simulink model "qdqd_robot"  (R2022b)
settings: Solver=FixedStepAuto  StartTime=0.0  StopTime=10  FixedStep=0.01  RelTol=1e-3
model workspace: external: MATLAB File C:\Users\Tin\Desktop\tailieuhoc\TT Robotics\task2\robot_DataFile2.m (data not in the file)
undefined symbols (not defined in the file or in its folder): smiData, X, Y, Z
libraries: sm_lib x21, nesl_utility x4
settings Model: Creator=Tin  LastModifiedBy=Tin

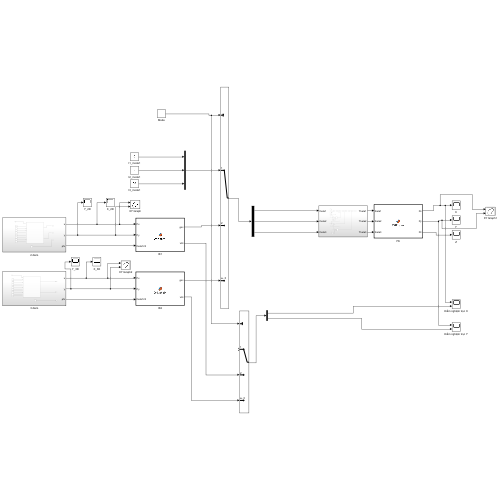
[thumbnail: Simulink's stored preview of the top-level diagram]
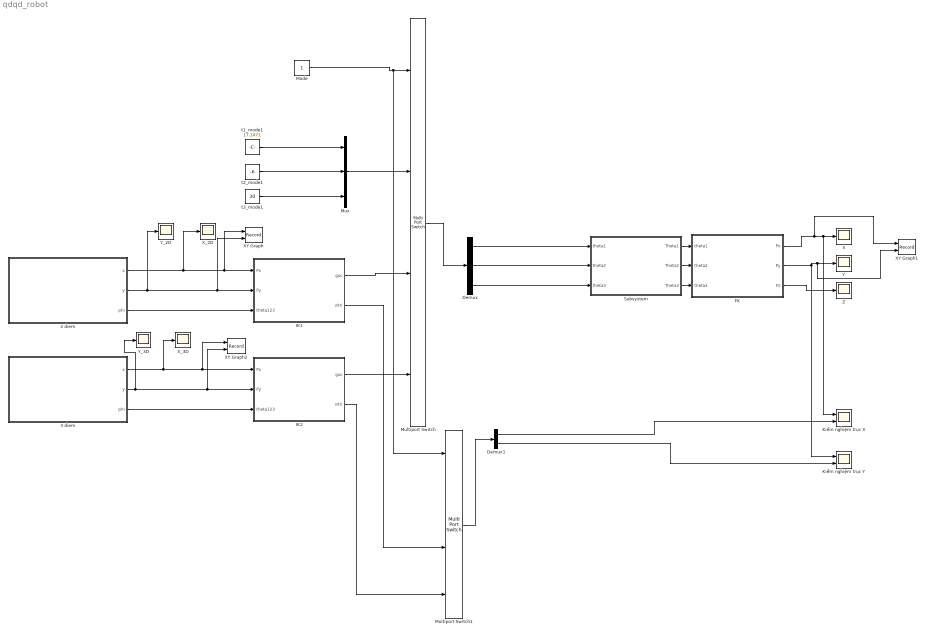
== system qdqd_robot ==
  2 diem : Subsystem
  3 diem : Subsystem
  Demux : Demux  Outputs=3
  Demux1 : Demux  Outputs=2
  FK : MATLAB Function  TreatAsAtomicUnit=on
  IK1 : MATLAB Function  TreatAsAtomicUnit=on
  IK2 : MATLAB Function  TreatAsAtomicUnit=on
  Kiểm nghiệm trục X : Scope  NumInputPorts=2
  Kiểm nghiệm trục Y : Scope  NumInputPorts=2
  Mode : Constant
  Multiport Switch : MultiPortSwitch  SaturateOnIntegerOverflow=off  InputSameDT=off
  Multiport Switch1 : MultiPortSwitch  SaturateOnIntegerOverflow=off  InputSameDT=off
  Mux : Mux  Inputs=3
  Subsystem : Subsystem
  X : Scope
  XY Graph : Record  FileSettingsInternal="{\"entries\":[{\"content\":{\"excelSettings\":{\"content\":{},\"type\":\"Streamout.ExcelSettings\"}},\"type\":\"Streamout.FileSettingStorage\",\"uuid\":\"97201033-76aa-4202-b919-b78145d5e60c\"}],\"packageUris\":[\"http://schema.mathworks.com/mf0/streamout_blocks/R2020a\"],\"version\":\"1.0\"}"  Layout=[1 1]  SignalsInternal="{\"entries\":[{\"content\":{\"signals\":[{\"content\":{\"blockPath\":[\"qdqd_robot/XY Graph\"],\"channel\":[],\"dimensions\":[1],\"domain\":\"qdqd_robot/XY Graph\",\"lineColor\":\"#a2142f\",\"plots\":[1],\"port\":1,\"sid\":[\"\"],\"signalID\":186,\"signalName\":\"2 diem:1\"},\"type\":\"RecordBlkView.Signal\",\"uuid\":\"08513785-76e9-4c55-b008-f54bb21082a6\"},{\"content\":{\"blockPath\":[\"qdqd_robot/XY Graph\"],\"channel\":[],\"dimensions\":[1],\"domain\":\"qdqd_robot/XY Graph\",\"lineColor\":\"#139fff\",\"plots\":[1],\"port\":2,\"sid\":[\"\"],\"signalID\":190,\"signalName\":\"2 diem:2\"},\"type\":\"RecordBlkView.Signal\",\"uuid\":\"6af3ea91-2b2f-4a9b-90b3-e45fbf568ca8\"}]},\"type\":\"RecordBlkView.InputSignals\",\"uuid\":\"c4f7b2ae-604a-40bb-aba8-63fb868da412\"}],\"packageUris\":[\"http://schema.mathworks.com/mf0/streamout_blocks/R2020a\"],\"version\":\"1.0\"}"  VisualizationBindings="{\"xyplotplugin\":{\"info\":[{\"series\":[{\"bindingParametersList\":[{\"parameter\":\"X-Axis\",\"signalID\":186,\"signalName\":\"2 diem:1\"},{\"parameter\":\"Y-Axis\",\"signalID\":190,\"signalName\":\"2 diem:2\"}],\"seriesID\":19907}],\"subplotID\":1}]}}"  CompatibilityTag=XY
  XY Graph1 : Record  FileSettingsInternal="{\"entries\":[{\"content\":{\"excelSettings\":{\"content\":{},\"type\":\"Streamout.ExcelSettings\"}},\"type\":\"Streamout.FileSettingStorage\",\"uuid\":\"ef5a2e5f-ada7-4355-a35d-416917ef2084\"}],\"packageUris\":[\"http://schema.mathworks.com/mf0/streamout_blocks/R2020a\"],\"version\":\"1.0\"}"  Layout=[1 1]  SignalsInternal="{\"entries\":[{\"content\":{\"signals\":[{\"content\":{\"blockPath\":[\"qdqd_robot/XY Graph1\"],\"channel\":[],\"dimensions\":[1],\"domain\":\"qdqd_robot/XY Graph1\",\"lineColor\":\"#a2142f\",\"plots\":[1],\"port\":1,\"sid\":[\"\"],\"signalID\":194,\"signalName\":\"FK:1\"},\"type\":\"RecordBlkView.Signal\",\"uuid\":\"117ca86f-aa11-44ab-9443-b09f4f7bf889\"},{\"content\":{\"blockPath\":[\"qdqd_robot/XY Graph1\"],\"channel\":[],\"dimensions\":[1],\"domain\":\"qdqd_robot/XY Graph1\",\"lineColor\":\"#139fff\",\"plots\":[1],\"port\":2,\"sid\":[\"\"],\"signalID\":198,\"signalName\":\"FK:2\"},\"type\":\"RecordBlkView.Signal\",\"uuid\":\"99251a9f-89e7-4e57-8cb5-748fe57cbdd2\"}]},\"type\":\"RecordBlkView.InputSignals\",\"uuid\":\"e90fa3b0-753d-4f20-842e-d0b0260bec66\"}],\"packageUris\":[\"http://schema.mathworks.com/mf0/streamout_blocks/R2020a\"],\"version\":\"1.0\"}"  VisualizationBindings="{\"xyplotplugin\":{\"info\":[{\"series\":[{\"bindingParametersList\":[{\"parameter\":\"X-Axis\",\"signalID\":194,\"signalName\":\"FK:1\"},{\"parameter\":\"Y-Axis\",\"signalID\":198,\"signalName\":\"FK:2\"}],\"seriesID\":49500}],\"subplotID\":1}]}}"  CompatibilityTag=XY
  XY Graph2 : Record  FileSettingsInternal="{\"entries\":[{\"content\":{\"excelSettings\":{\"content\":{},\"type\":\"Streamout.ExcelSettings\"}},\"type\":\"Streamout.FileSettingStorage\",\"uuid\":\"42d82971-a484-44fd-ac3b-312511253240\"}],\"packageUris\":[\"http://schema.mathworks.com/mf0/streamout_blocks/R2020a\"],\"version\":\"1.0\"}"  Layout=[1 1]  SignalsInternal="{\"entries\":[{\"content\":{\"signals\":[{\"content\":{\"blockPath\":[\"qdqd_robot/XY Graph2\"],\"channel\":[],\"dimensions\":[1],\"domain\":\"qdqd_robot/XY Graph2\",\"lineColor\":\"#a2142f\",\"plots\":[1],\"port\":1,\"sid\":[\"\"],\"signalID\":202,\"signalName\":\"3 diem:1\"},\"type\":\"RecordBlkView.Signal\",\"uuid\":\"d0b55c77-b964-4692-b3b0-299111d60012\"},{\"content\":{\"blockPath\":[\"qdqd_robot/XY Graph2\"],\"channel\":[],\"dimensions\":[1],\"domain\":\"qdqd_robot/XY Graph2\",\"lineColor\":\"#139fff\",\"plots\":[1],\"port\":2,\"sid\":[\"\"],\"signalID\":206,\"signalName\":\"3 diem:2\"},\"type\":\"RecordBlkView.Signal\",\"uuid\":\"4c5f2143-5546-468c-9f3f-87db4ee2b5a3\"}]},\"type\":\"RecordBlkView.InputSignals\",\"uuid\":\"6f2205dc-2759-4ab6-9096-b1192ef20588\"}],\"packageUris\":[\"http://schema.mathworks.com/mf0/streamout_blocks/R2020a\"],\"version\":\"1.0\"}"  VisualizationBindings="{\"xyplotplugin\":{\"info\":[{\"series\":[{\"bindingParametersList\":[{\"parameter\":\"X-Axis\",\"signalID\":202,\"signalName\":\"3 diem:1\"},{\"parameter\":\"Y-Axis\",\"signalID\":206,\"signalName\":\"3 diem:2\"}],\"seriesID\":60577}],\"subplotID\":1}]}}"  CompatibilityTag=XY
  X_2D : Scope
  X_3D : Scope
  Y : Scope
  Y_2D : Scope
  Y_3D : Scope
  Z : Scope
  t1_mode1 : Constant  Value=17.1471
  t2_mode1 : Constant  Value=-6
  t3_mode1 : Constant  Value=30
  wires:
  2 diem/3(phi) -> IK1/3(theta123)
  2 diem/2(y) -> Y_2D/1, IK1/2(Py), XY Graph/2
  3 diem/3(phi) -> IK2/3(theta123)
  IK2/1(goc) -> Multiport Switch/4
  t2_mode1/1 -> Mux/2
  t3_mode1/1 -> Mux/3
  Mux/1 -> Multiport Switch/2
  Demux/2 -> Subsystem/2(theta2)
  Demux/3 -> Subsystem/3(theta3)
  Multiport Switch/1 -> Demux/1
  t1_mode1/1 -> Mux/1
  3 diem/2(y) -> Y_3D/1, IK2/2(Py), XY Graph2/2
  3 diem/1(x) -> IK2/1(Px), XY Graph2/1, X_3D/1
  IK1/1(goc) -> Multiport Switch/3
  Subsystem/1(Theta1) -> FK/1(theta1)
  Subsystem/2(Theta2) -> FK/2(theta2)
  Subsystem/3(Theta3) -> FK/3(theta3)
  FK/1(Px) -> XY Graph1/1, Kiểm nghiệm trục X/1, X/1
  FK/2(Py) -> XY Graph1/2, Y/1, Kiểm nghiệm trục Y/1
  FK/3(Pz) -> Z/1
  Demux/1 -> Subsystem/1(theta1)
  2 diem/1(x) -> IK1/1(Px), XY Graph/1, X_2D/1
  Mode/1 -> Multiport Switch1/1, Multiport Switch/1
  IK1/2(vitri) -> Multiport Switch1/3
  IK2/2(vitri) -> Multiport Switch1/4
  Multiport Switch1/1 -> Demux1/1
  Demux1/1 -> Kiểm nghiệm trục X/2
  Demux1/2 -> Kiểm nghiệm trục Y/2

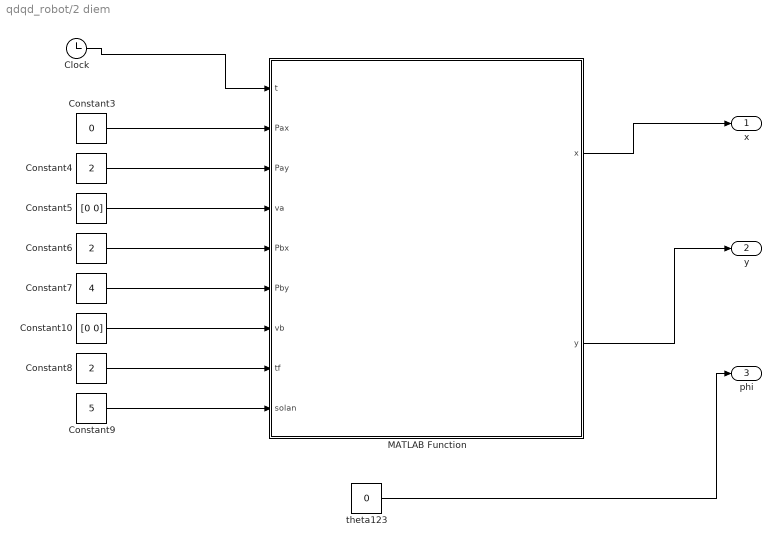
== system qdqd_robot/2 diem ==
  Clock : Clock
  Constant10 : Constant  Value=[0 0]
  Constant3 : Constant  Value=0
  Constant4 : Constant  Value=2
  Constant5 : Constant  Value=[0 0]
  Constant6 : Constant  Value=2
  Constant7 : Constant  Value=4
  Constant8 : Constant  Value=2
  Constant9 : Constant  Value=5
  MATLAB Function : MATLAB Function  TreatAsAtomicUnit=on
  theta123 : Constant  Value=0
  x : Outport
  y : Outport  Port=2
  phi : Outport  Port=3
  wires:
  Constant6/1 -> MATLAB Function/5(Pbx)
  Constant3/1 -> MATLAB Function/2(Pax)
  Constant7/1 -> MATLAB Function/6(Pby)
  Clock/1 -> MATLAB Function/1(t)
  Constant8/1 -> MATLAB Function/8(tf)
  Constant9/1 -> MATLAB Function/9(solan)
  Constant10/1 -> MATLAB Function/7(vb)
  Constant5/1 -> MATLAB Function/4(va)
  Constant4/1 -> MATLAB Function/3(Pay)
  MATLAB Function/1(x) -> x/1
  theta123/1 -> phi/1
  MATLAB Function/2(y) -> y/1

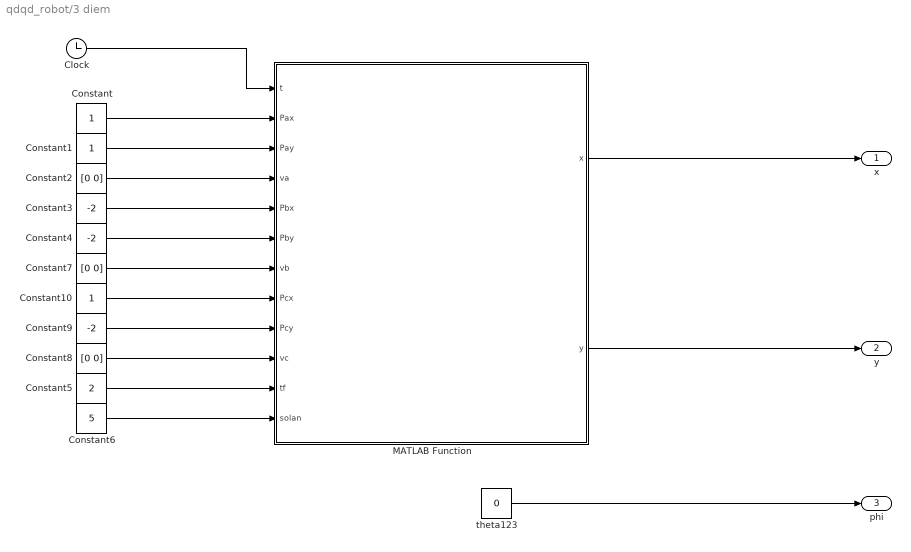
== system qdqd_robot/3 diem ==
  Clock : Clock
      settings: Decimation=30
  Constant : Constant
  Constant1 : Constant
  Constant10 : Constant
  Constant2 : Constant  Value=[0 0]
  Constant3 : Constant  Value=-2
  Constant4 : Constant  Value=-2
  Constant5 : Constant  Value=2
  Constant6 : Constant  Value=5
  Constant7 : Constant  Value=[0 0]
  Constant8 : Constant  Value=[0 0]
  Constant9 : Constant  Value=-2
  MATLAB Function : MATLAB Function  TreatAsAtomicUnit=on
  theta123 : Constant  Value=0
  x : Outport
  y : Outport  Port=2
  phi : Outport  Port=3
  wires:
  theta123/1 -> phi/1
  Constant10/1 -> MATLAB Function/8(Pcx)
  Constant9/1 -> MATLAB Function/9(Pcy)
  Constant3/1 -> MATLAB Function/5(Pbx)
  Constant8/1 -> MATLAB Function/10(vc)
  Constant5/1 -> MATLAB Function/11(tf)
  Constant/1 -> MATLAB Function/2(Pax)
  Constant2/1 -> MATLAB Function/4(va)
  Clock/1 -> MATLAB Function/1(t)
  Constant4/1 -> MATLAB Function/6(Pby)
  Constant1/1 -> MATLAB Function/3(Pay)
  Constant7/1 -> MATLAB Function/7(vb)
  Constant6/1 -> MATLAB Function/12(solan)
  MATLAB Function/1(x) -> x/1
  MATLAB Function/2(y) -> y/1

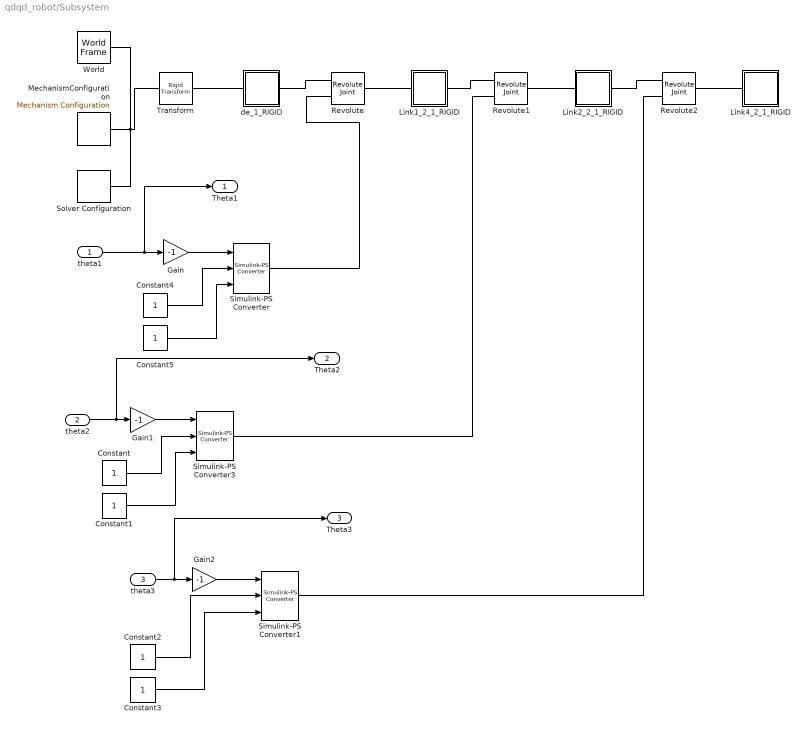
== system qdqd_robot/Subsystem ==
  theta1 : Inport
  theta2 : Inport  Port=2
  theta3 : Inport  Port=3
  Constant{,1..5} (6 alike) : Constant
  Gain : Gain  Gain=-1
  Gain1 : Gain  Gain=-1
  Gain2 : Gain  Gain=-1
  Link1_2_1_RIGID : Subsystem
  Link2_2_1_RIGID : Subsystem
  Link4_2_1_RIGID : Subsystem
  MechanismConfiguration : sm_lib/Utilities/Mechanism Configuration  UniformGravity=Constant  GravityVector=[0 -9.80665 0]  GravityUnits=m/s^2  LinearizationDelta=0.001  JointModeTransitionNonlinearIterations=2
  Revolute : sm_lib/Joints/Revolute Joint  JointMode=Normal  SenseConstraintForce=off  SenseConstraintForceX=off  SenseConstraintForceY=off  SenseConstraintForceZ=off  SenseConstraintTorque=off  SenseConstraintTorqueX=off  SenseConstraintTorqueY=off  SenseConstraintTorqueZ=off  SenseTotalForce=off  SenseTotalForceX=off  SenseTotalForceY=off  SenseTotalForceZ=off  SenseTotalTorque=off  SenseTotalTorqueX=off  SenseTotalTorqueY=off  SenseTotalTorqueZ=off  CompositeWrenchDir=FollowerOnBase  CompositeWrenchFrame=BaseFrame  EquilibriumPosition=0  EquilibriumPositionUnits=deg  SpringStiffness=0  SpringStiffnessUnits=N*m/deg  DampingCoefficient=0  DampingCoefficientUnits=N*m/(deg/s)  TorqueActuationMode=ComputedTorque  MotionActuationMode=InputMotion  SensePosition=off  SenseVelocity=off  SenseAcceleration=off  SenseTorqueForce=off  SenseLowerLimitTorqueForce=off  SenseUpperLimitTorqueForce=off  LowerLimitSpecify=off  LowerLimitBound=-90  LowerLimitBoundUnits=deg  LowerLimitStiffness=1e4  LowerLimitStiffnessUnits=N*m/deg  LowerLimitDamping=10  LowerLimitDampingUnits=N*m/(deg/s)  LowerLimitTransitionRegionWidth=0.1  LowerLimitTransitionRegionWidthUnits=deg  UpperLimitSpecify=off  UpperLimitBound=90  UpperLimitBoundUnits=deg  UpperLimitStiffness=1e4  UpperLimitStiffnessUnits=N*m/deg  UpperLimitDamping=10  UpperLimitDampingUnits=N*m/(deg/s)  UpperLimitTransitionRegionWidth=0.1  UpperLimitTransitionRegionWidthUnits=deg  PositionTargetSpecify=on  PositionTargetPriority=Low  PositionTargetValue=smiData.RevoluteJoint(1).Rz.Pos  PositionTargetValueUnits=deg  VelocityTargetSpecify=off  VelocityTargetPriority=High  VelocityTargetValue=0  VelocityTargetValueUnits=deg/s
  Revolute1 : sm_lib/Joints/Revolute Joint  JointMode=Normal  SenseConstraintForce=off  SenseConstraintForceX=off  SenseConstraintForceY=off  SenseConstraintForceZ=off  SenseConstraintTorque=off  SenseConstraintTorqueX=off  SenseConstraintTorqueY=off  SenseConstraintTorqueZ=off  SenseTotalForce=off  SenseTotalForceX=off  SenseTotalForceY=off  SenseTotalForceZ=off  SenseTotalTorque=off  SenseTotalTorqueX=off  SenseTotalTorqueY=off  SenseTotalTorqueZ=off  CompositeWrenchDir=FollowerOnBase  CompositeWrenchFrame=BaseFrame  EquilibriumPosition=0  EquilibriumPositionUnits=deg  SpringStiffness=0  SpringStiffnessUnits=N*m/deg  DampingCoefficient=0  DampingCoefficientUnits=N*m/(deg/s)  TorqueActuationMode=ComputedTorque  MotionActuationMode=InputMotion  SensePosition=off  SenseVelocity=off  SenseAcceleration=off  SenseTorqueForce=off  SenseLowerLimitTorqueForce=off  SenseUpperLimitTorqueForce=off  LowerLimitSpecify=off  LowerLimitBound=-90  LowerLimitBoundUnits=deg  LowerLimitStiffness=1e4  LowerLimitStiffnessUnits=N*m/deg  LowerLimitDamping=10  LowerLimitDampingUnits=N*m/(deg/s)  LowerLimitTransitionRegionWidth=0.1  LowerLimitTransitionRegionWidthUnits=deg  UpperLimitSpecify=off  UpperLimitBound=90  UpperLimitBoundUnits=deg  UpperLimitStiffness=1e4  UpperLimitStiffnessUnits=N*m/deg  UpperLimitDamping=10  UpperLimitDampingUnits=N*m/(deg/s)  UpperLimitTransitionRegionWidth=0.1  UpperLimitTransitionRegionWidthUnits=deg  PositionTargetSpecify=on  PositionTargetPriority=Low  PositionTargetValue=smiData.RevoluteJoint(2).Rz.Pos  PositionTargetValueUnits=deg  VelocityTargetSpecify=off  VelocityTargetPriority=High  VelocityTargetValue=0  VelocityTargetValueUnits=deg/s
  Revolute2 : sm_lib/Joints/Revolute Joint  JointMode=Normal  SenseConstraintForce=off  SenseConstraintForceX=off  SenseConstraintForceY=off  SenseConstraintForceZ=off  SenseConstraintTorque=off  SenseConstraintTorqueX=off  SenseConstraintTorqueY=off  SenseConstraintTorqueZ=off  SenseTotalForce=off  SenseTotalForceX=off  SenseTotalForceY=off  SenseTotalForceZ=off  SenseTotalTorque=off  SenseTotalTorqueX=off  SenseTotalTorqueY=off  SenseTotalTorqueZ=off  CompositeWrenchDir=FollowerOnBase  CompositeWrenchFrame=BaseFrame  EquilibriumPosition=0  EquilibriumPositionUnits=deg  SpringStiffness=0  SpringStiffnessUnits=N*m/deg  DampingCoefficient=0  DampingCoefficientUnits=N*m/(deg/s)  TorqueActuationMode=ComputedTorque  MotionActuationMode=InputMotion  SensePosition=off  SenseVelocity=off  SenseAcceleration=off  SenseTorqueForce=off  SenseLowerLimitTorqueForce=off  SenseUpperLimitTorqueForce=off  LowerLimitSpecify=off  LowerLimitBound=-90  LowerLimitBoundUnits=deg  LowerLimitStiffness=1e4  LowerLimitStiffnessUnits=N*m/deg  LowerLimitDamping=10  LowerLimitDampingUnits=N*m/(deg/s)  LowerLimitTransitionRegionWidth=0.1  LowerLimitTransitionRegionWidthUnits=deg  UpperLimitSpecify=off  UpperLimitBound=90  UpperLimitBoundUnits=deg  UpperLimitStiffness=1e4  UpperLimitStiffnessUnits=N*m/deg  UpperLimitDamping=10  UpperLimitDampingUnits=N*m/(deg/s)  UpperLimitTransitionRegionWidth=0.1  UpperLimitTransitionRegionWidthUnits=deg  PositionTargetSpecify=on  PositionTargetPriority=Low  PositionTargetValue=smiData.RevoluteJoint(3).Rz.Pos  PositionTargetValueUnits=deg  VelocityTargetSpecify=off  VelocityTargetPriority=High  VelocityTargetValue=0  VelocityTargetValueUnits=deg/s
  Simulink-PS Converter : nesl_utility/Simulink-PS Converter  PhysicalDomain=network_engine_domain  SubClassName=ps_input  LeftPortType=input  RightPortType=output  PseudoPeriodic=off  Frequencies=[]  NoiseDistribution=none  NoiseParameters=[]  Unit=1  AffineConversion=on  FilteringAndDerivatives=provide  SimscapeFilterOrder=2  InputFilterTimeConstant=0.001  UdotUserProvided=2
  Simulink-PS Converter1 : nesl_utility/Simulink-PS Converter  PhysicalDomain=network_engine_domain  SubClassName=ps_input  LeftPortType=input  RightPortType=output  PseudoPeriodic=off  Frequencies=[]  NoiseDistribution=none  NoiseParameters=[]  Unit=1  AffineConversion=on  FilteringAndDerivatives=provide  SimscapeFilterOrder=2  InputFilterTimeConstant=0.001  UdotUserProvided=2
  Simulink-PS Converter3 : nesl_utility/Simulink-PS Converter  PhysicalDomain=network_engine_domain  SubClassName=ps_input  LeftPortType=input  RightPortType=output  PseudoPeriodic=off  Frequencies=[]  NoiseDistribution=none  NoiseParameters=[]  Unit=1  AffineConversion=on  FilteringAndDerivatives=provide  SimscapeFilterOrder=2  InputFilterTimeConstant=0.001  UdotUserProvided=2
  Solver Configuration : nesl_utility/Solver Configuration  PhysicalDomain=network_engine_domain  SubClassName=solver  LeftPortType=input  RightPortType=generic  Tones=[]  Harmonics=[]  SimulateNoise=off  Profile=off  UseLocalSampling=off  EnableSwitchedLinearOptims=on  FrequencyDomain=off  UseCCode=off  RelTol=0.001  AbsTol=0.001  MinStep=1e-09  ToWorkspace=off  RevertToSquareIcSolve=off  NumHomotopyIterations=100  PhasorMode=off  PhasorModeNumHarmonics=1  ConsistencySolver=NEWTON_XTOL_AFTER_FTOL  IndexReductionMethod=DerivativeReplacement  DoDC=off  ResidualTolerance=1e-09  ConsistencyTolSource=GLOBAL  ConsistencyAbsTol=0.001  ConsistencyRelTol=0.001  ConsistencyTolFactor=0.001  UseLocalSolver=off  LocalSolverChoice=NE_BACKWARD_EULER_ADVANCER  ResolveIndetEquations=on  FunctionEvalNumThread=1  LocalSolverSampleTime=0.001  DoFixedCost=off  MaxNonlinIter=3  MaxModeIter=2  ComputeImpulses=off  ImpulseIterations=2  LinearAlgebra=auto  LinearAlgebraNumThread=0  EquationFormulation=NE_TIME_EF  DelaysMemoryBudget=1024  AutomaticFiltering=on  FilteringTimeConstant=0.001  PartitionStorageMethod=AS_NEEDED  PartitionMemoryBudget=1024  PartitionMethod=ROBUST
  Transform : sm_lib/Frames and Transforms/Rigid Transform  TranslationMethod=Cartesian  TranslationStandardOffset=0  TranslationLengthUnit=mm  TranslationStandardAxis=+Z  TranslationCartesianOffset=smiData.RigidTransform(2).translation  TranslationROffset=0  TranslationROffsetUnits=m  TranslationZOffset=0  TranslationZOffsetUnits=m  TranslationThetaOffset=0  TranslationThetaOffsetUnits=deg  RotationMethod=ArbitraryAxis  RotationAngleUnits=rad  RotationStandardAxis=+Z  RotationAngle=smiData.RigidTransform(2).angle  RotationArbitraryAxis=smiData.RigidTransform(2).axis  FollAlignAxisA=+X  BaseAlignAxisA=+Y  FollAlignAxisB=+Y  BaseAlignAxisB=+Z  RotationSequenceAxes=FollowerAxes  RotationSequence=XYX  RotationSequenceAngles=[0 0 0]  RotationSequenceAnglesUnits=deg  RotationMatrix=[1 0 0; 0 1 0; 0 0 1]  Quaternion=[1 0 0 0]
  World : sm_lib/Frames and Transforms/World Frame
  de_1_RIGID : Subsystem
  Theta1 : Outport
  Theta2 : Outport  Port=2
  Theta3 : Outport  Port=3
  wires:
  theta2/1 -> Theta2/1, Gain1/1
  Gain1/1 -> Simulink-PS Converter3/1
  Gain2/1 -> Simulink-PS Converter1/1
  theta3/1 -> Theta3/1, Gain2/1
  Constant/1 -> Simulink-PS Converter3/2
  Constant1/1 -> Simulink-PS Converter3/3
  Constant2/1 -> Simulink-PS Converter1/2
  Constant3/1 -> Simulink-PS Converter1/3
  Constant4/1 -> Simulink-PS Converter/2
  Constant5/1 -> Simulink-PS Converter/3
  Gain/1 -> Simulink-PS Converter/1
  theta1/1 -> Theta1/1, Gain/1
  connections:
  World/RConn1 -- MechanismConfiguration/RConn1 -- Solver Configuration/RConn1 -- Transform/LConn1
  Simulink-PS Converter/RConn1 -- Revolute/LConn2
  Link1_2_1_RIGID/LConn1 -- Revolute/RConn1
  Link2_2_1_RIGID/RConn1 -- Revolute2/LConn1
  Transform/RConn1 -- de_1_RIGID/LConn1
  Link2_2_1_RIGID/LConn1 -- Revolute1/RConn1
  Link4_2_1_RIGID/LConn1 -- Revolute2/RConn1
  Revolute/LConn1 -- de_1_RIGID/RConn1
  Link1_2_1_RIGID/RConn1 -- Revolute1/LConn1
  Revolute1/LConn2 -- Simulink-PS Converter3/RConn1
  Simulink-PS Converter1/RConn1 -- Revolute2/LConn2

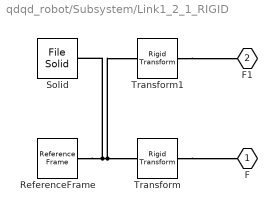
== system qdqd_robot/Subsystem/Link1_2_1_RIGID ==
  ReferenceFrame : sm_lib/Frames and Transforms/Reference Frame
  Solid : sm_lib/Body Elements/File Solid  ExtGeomFileName=C:\Users\Tin\Desktop\tailieuhoc\TT Robotics\task2\Link1_2_Default_sldprt.STEP  UnitType=FromFile  ExtGeomFileUnits=m  StepReaderType=HEX  ExportConvexHullGeometry=off  InertiaType=Custom  Mass=smiData.Solid(3).mass  MassUnits=kg  CenterOfMass=smiData.Solid(3).CoM  CenterOfMassUnits=mm  MomentsOfInertia=smiData.Solid(3).MoI  MomentsOfInertiaUnits=kg*mm^2  ProductsOfInertia=smiData.Solid(3).PoI  ProductsOfInertiaUnits=kg*mm^2  BasedOnType=DensityFromFile  Density=1000  DensityUnits=kg/m^3  DoExposeReferenceFrame=on  SerializedFrames=<Frames/>  GraphicType=FromGeometry  MarkerShape=Sphere  MarkerSize=10  GraphicVisPropType=SimpleVisualProperties  GraphicDiffuseColor=smiData.Solid(3).color  GraphicSpecularColor=[0.5 0.5 0.5 1.0]  GraphicAmbientColor=[0.15 0.15 0.15 1.0]  GraphicEmissiveColor=[0.0 0.0 0.0 1.0]  GraphicShininess=75  GraphicOpacity=smiData.Solid(3).opacity
  Transform : sm_lib/Frames and Transforms/Rigid Transform  TranslationMethod=Cartesian  TranslationStandardOffset=0  TranslationLengthUnit=mm  TranslationStandardAxis=+Z  TranslationCartesianOffset=smiData.RigidTransform(4).translation  TranslationROffset=0  TranslationROffsetUnits=m  TranslationZOffset=0  TranslationZOffsetUnits=m  TranslationThetaOffset=0  TranslationThetaOffsetUnits=deg  RotationMethod=ArbitraryAxis  RotationAngleUnits=rad  RotationStandardAxis=+Z  RotationAngle=smiData.RigidTransform(4).angle  RotationArbitraryAxis=smiData.RigidTransform(4).axis  FollAlignAxisA=+X  BaseAlignAxisA=+Y  FollAlignAxisB=+Y  BaseAlignAxisB=+Z  RotationSequenceAxes=FollowerAxes  RotationSequence=XYX  RotationSequenceAngles=[0 0 0]  RotationSequenceAnglesUnits=deg  RotationMatrix=[1 0 0; 0 1 0; 0 0 1]  Quaternion=[1 0 0 0]
  Transform1 : sm_lib/Frames and Transforms/Rigid Transform  TranslationMethod=Cartesian  TranslationStandardOffset=0  TranslationLengthUnit=mm  TranslationStandardAxis=+Z  TranslationCartesianOffset=smiData.RigidTransform(5).translation  TranslationROffset=0  TranslationROffsetUnits=m  TranslationZOffset=0  TranslationZOffsetUnits=m  TranslationThetaOffset=0  TranslationThetaOffsetUnits=deg  RotationMethod=ArbitraryAxis  RotationAngleUnits=rad  RotationStandardAxis=+Z  RotationAngle=smiData.RigidTransform(5).angle  RotationArbitraryAxis=smiData.RigidTransform(5).axis  FollAlignAxisA=+X  BaseAlignAxisA=+Y  FollAlignAxisB=+Y  BaseAlignAxisB=+Z  RotationSequenceAxes=FollowerAxes  RotationSequence=XYX  RotationSequenceAngles=[0 0 0]  RotationSequenceAnglesUnits=deg  RotationMatrix=[1 0 0; 0 1 0; 0 0 1]  Quaternion=[1 0 0 0]
  F : PMIOPort  Side=Left
  F1 : PMIOPort  Port=2  Side=Right
  connections:
  ReferenceFrame/RConn1 -- Transform/LConn1 -- Transform1/LConn1 -- Solid/RConn1
  Transform/RConn1 -- F/RConn1
  Transform1/RConn1 -- F1/RConn1

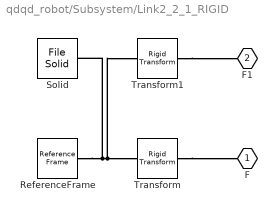
== system qdqd_robot/Subsystem/Link2_2_1_RIGID ==
  ReferenceFrame : sm_lib/Frames and Transforms/Reference Frame
  Solid : sm_lib/Body Elements/File Solid  ExtGeomFileName=C:\Users\Tin\Desktop\tailieuhoc\TT Robotics\task2\Link2_2_Default_sldprt.STEP  UnitType=FromFile  ExtGeomFileUnits=m  StepReaderType=HEX  ExportConvexHullGeometry=off  InertiaType=Custom  Mass=smiData.Solid(4).mass  MassUnits=kg  CenterOfMass=smiData.Solid(4).CoM  CenterOfMassUnits=mm  MomentsOfInertia=smiData.Solid(4).MoI  MomentsOfInertiaUnits=kg*mm^2  ProductsOfInertia=smiData.Solid(4).PoI  ProductsOfInertiaUnits=kg*mm^2  BasedOnType=DensityFromFile  Density=1000  DensityUnits=kg/m^3  DoExposeReferenceFrame=on  SerializedFrames=<Frames/>  GraphicType=FromGeometry  MarkerShape=Sphere  MarkerSize=10  GraphicVisPropType=SimpleVisualProperties  GraphicDiffuseColor=smiData.Solid(4).color  GraphicSpecularColor=[0.5 0.5 0.5 1.0]  GraphicAmbientColor=[0.15 0.15 0.15 1.0]  GraphicEmissiveColor=[0.0 0.0 0.0 1.0]  GraphicShininess=75  GraphicOpacity=smiData.Solid(4).opacity
  Transform : sm_lib/Frames and Transforms/Rigid Transform  TranslationMethod=Cartesian  TranslationStandardOffset=0  TranslationLengthUnit=mm  TranslationStandardAxis=+Z  TranslationCartesianOffset=smiData.RigidTransform(6).translation  TranslationROffset=0  TranslationROffsetUnits=m  TranslationZOffset=0  TranslationZOffsetUnits=m  TranslationThetaOffset=0  TranslationThetaOffsetUnits=deg  RotationMethod=ArbitraryAxis  RotationAngleUnits=rad  RotationStandardAxis=+Z  RotationAngle=smiData.RigidTransform(6).angle  RotationArbitraryAxis=smiData.RigidTransform(6).axis  FollAlignAxisA=+X  BaseAlignAxisA=+Y  FollAlignAxisB=+Y  BaseAlignAxisB=+Z  RotationSequenceAxes=FollowerAxes  RotationSequence=XYX  RotationSequenceAngles=[0 0 0]  RotationSequenceAnglesUnits=deg  RotationMatrix=[1 0 0; 0 1 0; 0 0 1]  Quaternion=[1 0 0 0]
  Transform1 : sm_lib/Frames and Transforms/Rigid Transform  TranslationMethod=Cartesian  TranslationStandardOffset=0  TranslationLengthUnit=mm  TranslationStandardAxis=+Z  TranslationCartesianOffset=smiData.RigidTransform(7).translation  TranslationROffset=0  TranslationROffsetUnits=m  TranslationZOffset=0  TranslationZOffsetUnits=m  TranslationThetaOffset=0  TranslationThetaOffsetUnits=deg  RotationMethod=ArbitraryAxis  RotationAngleUnits=rad  RotationStandardAxis=+Z  RotationAngle=smiData.RigidTransform(7).angle  RotationArbitraryAxis=smiData.RigidTransform(7).axis  FollAlignAxisA=+X  BaseAlignAxisA=+Y  FollAlignAxisB=+Y  BaseAlignAxisB=+Z  RotationSequenceAxes=FollowerAxes  RotationSequence=XYX  RotationSequenceAngles=[0 0 0]  RotationSequenceAnglesUnits=deg  RotationMatrix=[1 0 0; 0 1 0; 0 0 1]  Quaternion=[1 0 0 0]
  F : PMIOPort  Side=Left
  F1 : PMIOPort  Port=2  Side=Right
  connections:
  ReferenceFrame/RConn1 -- Transform/LConn1 -- Transform1/LConn1 -- Solid/RConn1
  Transform/RConn1 -- F/RConn1
  Transform1/RConn1 -- F1/RConn1

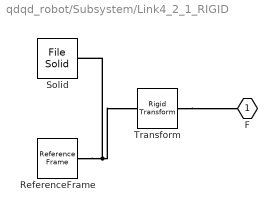
== system qdqd_robot/Subsystem/Link4_2_1_RIGID ==
  ReferenceFrame : sm_lib/Frames and Transforms/Reference Frame
  Solid : sm_lib/Body Elements/File Solid  ExtGeomFileName=C:\Users\Tin\Desktop\tailieuhoc\TT Robotics\task2\Link4_2_Default_sldprt.STEP  UnitType=FromFile  ExtGeomFileUnits=m  StepReaderType=HEX  ExportConvexHullGeometry=off  InertiaType=Custom  Mass=smiData.Solid(1).mass  MassUnits=kg  CenterOfMass=smiData.Solid(1).CoM  CenterOfMassUnits=mm  MomentsOfInertia=smiData.Solid(1).MoI  MomentsOfInertiaUnits=kg*mm^2  ProductsOfInertia=smiData.Solid(1).PoI  ProductsOfInertiaUnits=kg*mm^2  BasedOnType=DensityFromFile  Density=1000  DensityUnits=kg/m^3  DoExposeReferenceFrame=on  SerializedFrames=<Frames/>  GraphicType=FromGeometry  MarkerShape=Sphere  MarkerSize=10  GraphicVisPropType=SimpleVisualProperties  GraphicDiffuseColor=smiData.Solid(1).color  GraphicSpecularColor=[0.5 0.5 0.5 1.0]  GraphicAmbientColor=[0.15 0.15 0.15 1.0]  GraphicEmissiveColor=[0.0 0.0 0.0 1.0]  GraphicShininess=75  GraphicOpacity=smiData.Solid(1).opacity
  Transform : sm_lib/Frames and Transforms/Rigid Transform  TranslationMethod=Cartesian  TranslationStandardOffset=0  TranslationLengthUnit=mm  TranslationStandardAxis=+Z  TranslationCartesianOffset=smiData.RigidTransform(8).translation  TranslationROffset=0  TranslationROffsetUnits=m  TranslationZOffset=0  TranslationZOffsetUnits=m  TranslationThetaOffset=0  TranslationThetaOffsetUnits=deg  RotationMethod=ArbitraryAxis  RotationAngleUnits=rad  RotationStandardAxis=+Z  RotationAngle=smiData.RigidTransform(8).angle  RotationArbitraryAxis=smiData.RigidTransform(8).axis  FollAlignAxisA=+X  BaseAlignAxisA=+Y  FollAlignAxisB=+Y  BaseAlignAxisB=+Z  RotationSequenceAxes=FollowerAxes  RotationSequence=XYX  RotationSequenceAngles=[0 0 0]  RotationSequenceAnglesUnits=deg  RotationMatrix=[1 0 0; 0 1 0; 0 0 1]  Quaternion=[1 0 0 0]
  F : PMIOPort  Side=Left
  connections:
  ReferenceFrame/RConn1 -- Solid/RConn1 -- Transform/LConn1
  Transform/RConn1 -- F/RConn1

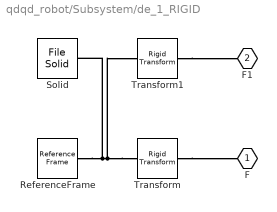
== system qdqd_robot/Subsystem/de_1_RIGID ==
  ReferenceFrame : sm_lib/Frames and Transforms/Reference Frame
  Solid : sm_lib/Body Elements/File Solid  ExtGeomFileName=C:\Users\Tin\Desktop\tailieuhoc\TT Robotics\task2\de_Default_sldprt.STEP  UnitType=FromFile  ExtGeomFileUnits=m  StepReaderType=HEX  ExportConvexHullGeometry=off  InertiaType=Custom  Mass=smiData.Solid(2).mass  MassUnits=kg  CenterOfMass=smiData.Solid(2).CoM  CenterOfMassUnits=mm  MomentsOfInertia=smiData.Solid(2).MoI  MomentsOfInertiaUnits=kg*mm^2  ProductsOfInertia=smiData.Solid(2).PoI  ProductsOfInertiaUnits=kg*mm^2  BasedOnType=DensityFromFile  Density=1000  DensityUnits=kg/m^3  DoExposeReferenceFrame=on  SerializedFrames=<Frames/>  GraphicType=FromGeometry  MarkerShape=Sphere  MarkerSize=10  GraphicVisPropType=SimpleVisualProperties  GraphicDiffuseColor=smiData.Solid(2).color  GraphicSpecularColor=[0.5 0.5 0.5 1.0]  GraphicAmbientColor=[0.15 0.15 0.15 1.0]  GraphicEmissiveColor=[0.0 0.0 0.0 1.0]  GraphicShininess=75  GraphicOpacity=smiData.Solid(2).opacity
  Transform : sm_lib/Frames and Transforms/Rigid Transform  TranslationMethod=Cartesian  TranslationStandardOffset=0  TranslationLengthUnit=mm  TranslationStandardAxis=+Z  TranslationCartesianOffset=smiData.RigidTransform(1).translation  TranslationROffset=0  TranslationROffsetUnits=m  TranslationZOffset=0  TranslationZOffsetUnits=m  TranslationThetaOffset=0  TranslationThetaOffsetUnits=deg  RotationMethod=ArbitraryAxis  RotationAngleUnits=rad  RotationStandardAxis=+Z  RotationAngle=smiData.RigidTransform(1).angle  RotationArbitraryAxis=smiData.RigidTransform(1).axis  FollAlignAxisA=+X  BaseAlignAxisA=+Y  FollAlignAxisB=+Y  BaseAlignAxisB=+Z  RotationSequenceAxes=FollowerAxes  RotationSequence=XYX  RotationSequenceAngles=[0 0 0]  RotationSequenceAnglesUnits=deg  RotationMatrix=[1 0 0; 0 1 0; 0 0 1]  Quaternion=[1 0 0 0]
  Transform1 : sm_lib/Frames and Transforms/Rigid Transform  TranslationMethod=Cartesian  TranslationStandardOffset=0  TranslationLengthUnit=mm  TranslationStandardAxis=+Z  TranslationCartesianOffset=smiData.RigidTransform(3).translation  TranslationROffset=0  TranslationROffsetUnits=m  TranslationZOffset=0  TranslationZOffsetUnits=m  TranslationThetaOffset=0  TranslationThetaOffsetUnits=deg  RotationMethod=ArbitraryAxis  RotationAngleUnits=rad  RotationStandardAxis=+Z  RotationAngle=smiData.RigidTransform(3).angle  RotationArbitraryAxis=smiData.RigidTransform(3).axis  FollAlignAxisA=+X  BaseAlignAxisA=+Y  FollAlignAxisB=+Y  BaseAlignAxisB=+Z  RotationSequenceAxes=FollowerAxes  RotationSequence=XYX  RotationSequenceAngles=[0 0 0]  RotationSequenceAnglesUnits=deg  RotationMatrix=[1 0 0; 0 1 0; 0 0 1]  Quaternion=[1 0 0 0]
  F : PMIOPort  Side=Left
  F1 : PMIOPort  Port=2  Side=Right
  connections:
  Transform/LConn1 -- Transform1/LConn1 -- ReferenceFrame/RConn1 -- Solid/RConn1
  Transform/RConn1 -- F/RConn1
  Transform1/RConn1 -- F1/RConn1

== matlab function qdqd_robot/IK1 ==
  data: Px input; goc output; Py input; theta123 input; vitri output
function [goc, vitri] = DHNghich(Px, Py, theta123)
    l1 = 100;
    l2 = 250;
    l3 = 250;
    l4 = 150;
    %tinh theta2
    nx = Px - l1 -l4*cosd(theta123);
    ny = Py - l4*sind(theta123);
    theta2 = atan2d (sqrt(1 - ((nx^2 + ny^2 - l2^2 - l3^2) / (2 * l2 * l3))^2), (nx^2 + ny^2 - l2^2 - l3^2) / (2 * l2 * l3));

    %tinh theta1
    A1 = ny * (l2 + l3 * cosd(theta2)) - l3*sind(theta2)*nx;
    A2 = (l2 + l3*cosd(theta2))^2 + (l3*sind(theta2))^2;
    A = A1/A2;

    B = (nx + l3*sind(theta2)*A) / (l2 + l3*cosd(theta2));
    theta1 = atan2d(A, B);
    %tinh theta3
    theta3 = theta123 - (theta2 + theta1);
    goc = [theta1; theta2; theta3];
    vitri = [Px; Py];
end

== matlab function qdqd_robot/2 diem/MATLAB Function ==
  data: x output; t input; y output; Pax input; Pay input; va input; Pbx input; Pby input; vb input; tf input; solan input
function [x, y] = QHQD2D(t, Pax, Pay, va, Pbx, Pby, vb, tf, solan)

    function [x, y] = TrajectoryPlanning(t, P0, v0, Pf, vf, tf, t0)
        a10 = P0(1);
        a20 = P0(2);
        a11 = v0(1);
        a21 = v0(2);  
    
        a12 = 3 / tf^2 * (Pf(1) - P0(1)) - 2 / tf * v0(1) - 1 / tf * vf(1);
        a22 = 3 / tf^2 * (Pf(2) - P0(2)) - 2 / tf * v0(2) - 1 / tf * vf(2);
        a13 = -2 / tf^3 * (Pf(1) - P0(1)) + 1 / tf^2 * (vf(1) + v0(1));
        a23 = -2 / tf^3 * (Pf(2) - P0(2)) + 1 / tf^2 * (vf(2) + v0(2));
    
        x = a10 + a11 *(t - t0) + a12 * (t - t0)^2 + a13*(t - t0)^3;
        y = a20 + a21 *(t - t0) + a22 * (t - t0)^2 + a23*(t - t0)^3;
    end

    chuky = tf*2;
    i = fix(t/chuky);
    Pa = [Pax Pay];
    Pb = [Pbx Pby];
    if(t <= (tf + chuky*i))
        [x, y] = TrajectoryPlanning(t, Pa, va, Pb, vb, tf, 0 + chuky * i);
    else
        [x, y] = TrajectoryPlanning(t, Pa, va, Pb, vb, tf, tf + chuky * i);
    end
    if(t > chuky*solan)
         x = Pax;
         y = Pay;
    end
end

== matlab function qdqd_robot/3 diem/MATLAB Function ==
  data: x output; t input; y output; Pax input; Pay input; va input; Pbx input; Pby input; vb input; Pcx input; Pcy input; vc input; tf input; solan input
function [x, y] = QHQD3D(t, Pax, Pay, va, Pbx, Pby, vb, Pcx, Pcy, vc, tf, solan) 
    function [x, y, z] = TrajectoryPlanning(t, P0, v0, Pf, vf, tf, t0)
        a10 = P0(1);
        a20 = P0(2);
        a11 = v0(1);
        a21 = v0(2);  
    
        a12 = 3 / tf^2 * (Pf(1) - P0(1)) - 2 / tf * v0(1) - 1 / tf * vf(1);
        a22 = 3 / tf^2 * (Pf(2) - P0(2)) - 2 / tf * v0(2) - 1 / tf * vf(2);
        a13 = -2 / tf^3 * (Pf(1) - P0(1)) + 1 / tf^2 * (vf(1) + v0(1));
        a23 = -2 / tf^3 * (Pf(2) - P0(2)) + 1 / tf^2 * (vf(2) + v0(2));
    
        x = a10 + a11 *(t - t0) + a12 * (t - t0)^2 + a13*(t - t0)^3;
        y = a20 + a21 *(t - t0) + a22 * (t - t0)^2 + a23*(t - t0)^3;
        z = 0;
    end
    chuky = tf*3;
    i = fix(t/chuky);
    Pa = [Pax Pay];
    Pb = [Pbx Pby];
    Pc = [Pcx Pcy];
    if(t <= (tf + chuky*i))
        [x, y] = TrajectoryPlanning(t, Pa, va, Pb, vb, tf, tf*0 + chuky * i);
    elseif(t <= (tf*2 + chuky*i))
        [x, y] = TrajectoryPlanning(t, Pb, vb, Pc, vc, tf, tf*1 + chuky * i);
    else
        [x, y] = TrajectoryPlanning(t, Pc, vc, Pa, va, tf, tf*2 + chuky * i);
    end
    if(t > chuky*solan)
         x = Pax;
         y = Pay;
    end
end

== matlab function qdqd_robot/IK2 ==
  data: Px input; goc output; Py input; theta123 input; vitri output
function [goc, vitri] = DHNghich(Px, Py, theta123)
    l1 = 100;
    l2 = 250;
    l3 = 250;
    l4 = 150;
    %tinh theta2
    nx = Px - l1 -l4*cosd(theta123);
    ny = Py - l4*sind(theta123);
    theta2 = atan2d (sqrt(1 - ((nx^2 + ny^2 - l2^2 - l3^2) / (2 * l2 * l3))^2), (nx^2 + ny^2 - l2^2 - l3^2) / (2 * l2 * l3));

    %tinh theta1
    A1 = ny * (l2 + l3 * cosd(theta2)) - l3*sind(theta2)*nx;
    A2 = (l2 + l3*cosd(theta2))^2 + (l3*sind(theta2))^2;
    A = A1/A2;

    B = (nx + l3*sind(theta2)*A) / (l2 + l3*cosd(theta2));
    theta1 = atan2d(A, B);
    %tinh theta3
    theta3 = theta123 - (theta2 + theta1);
    goc = [theta1; theta2; theta3];
    vitri = [Px; Py];
end

== matlab function qdqd_robot/FK ==
  data: theta1 input; Px output; theta2 input; theta3 input; Py output; Pz output
function [Px, Py, Pz] = DHThuan(theta1, theta2, theta3)
    l1 = 100;
    l2 = 250;
    l3 = 250;
    l4 = 150;
    d1 = 30;
    d2 = 30;
    d3 = 30;
    l0 = 150;
    theta123= theta1 + theta2 + theta3;
    Px = l1 + l2*cosd(theta1) + l3*cosd(theta1 + theta2) + l4*cosd(theta123);
    Py = l2*sind(theta1) + l3*sind(theta1 + theta2) + l4*sind(theta123);
    Pz = l0 + d1 + d2 + d3;
end
